simulink subsystem "Odometria"  (R2023b)
settings: Solver=VariableStepAuto  StartTime=0.0  StopTime=10.0  RelTol=1e-3
undefined symbols (not defined in the file): DiscIntNeverNeededParam
settings Model: Creator=Usuario_UMA  LastModifiedBy=Diego

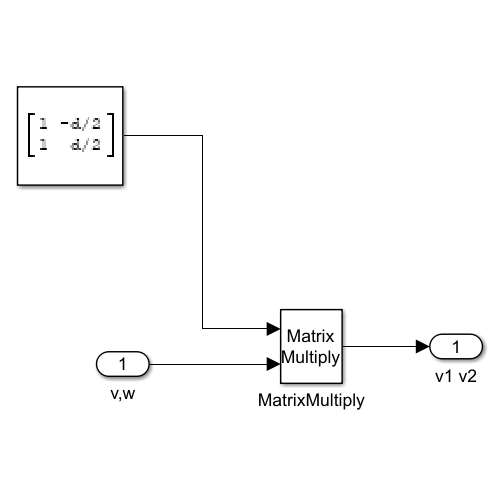
[thumbnail: Simulink's stored preview of the top-level diagram]
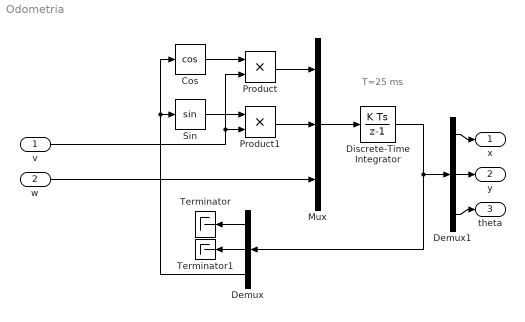
== system Odometria ==
  note: T=25 ms
  v : Inport
  w : Inport  Port=2
  Cos : Trigonometry  Operator=cos
  Demux : Demux  Outputs=3
  Demux1 : Demux  Outputs=3
  Discrete-Time Integrator : DiscreteIntegrator  SampleTime=25/1000  ICPrevOutput=DiscIntNeverNeededParam  ICPrevScaledInput=DiscIntNeverNeededParam
  Mux : Mux  Inputs=3
  Product : Product
  Product1 : Product
  Sin : Trigonometry
  Terminator : Terminator
  Terminator1 : Terminator
  x : Outport
  y : Outport  Port=2
  theta : Outport  Port=3
  wires:
  Discrete-Time Integrator/1 -> Demux1/1, Demux/1
  Demux/1 -> Terminator/1
  Demux/2 -> Terminator1/1
  Demux/3 -> Sin/1, Cos/1
  Cos/1 -> Product/1
  Sin/1 -> Product1/1
  v/1 -> Product1/2, Product/2
  w/1 -> Mux/3
  Product/1 -> Mux/1
  Product1/1 -> Mux/2
  Mux/1 -> Discrete-Time Integrator/1
  Demux1/1 -> x/1
  Demux1/2 -> y/1
  Demux1/3 -> theta/1
